simulink model "UPSControl"  (R2025b)
settings: Solver=VariableStepAuto  StartTime=0.0  StopTime=10  FixedStep=Ts  RelTol=1e-3
PostLoadFcn:
  | DataCenterParam;
values from neighbouring files (symbols this model uses):
  generator = struct    [GeneratorParam.m]
  lineInductance = 1e-6    (= 1e-06)    [DataCenterParam.m]    (also in GridParam.m)
  lineResistance = 1e-3    (= 0.001)    [DataCenterParam.m]    (also in GridParam.m)
  loadPower = 5e6    (= 5000000)    [DataCenterParam.m]    (also in LVRT.m; RedundancyAnalysis.m = 10000000)
  machine = struct    [GeneratorParam.m]
  powerTau = 0.005    [DataCenterParam.m]
  Ts = 5e-5    (= 5e-05)    [DataCenterParam.m]    (also in GeneratorParam.m)
  utilizationFactor = 0.45    [DataCenterParam.m]    (also in RedundancyAnalysis.m)
undefined symbols (not defined in the file or in its folder): breaker, ctLimitDelayTime, DiscIntNeverNeededParam, ee_sli_rtmsupport, gcbh, grid, rack, ups
libraries: nesl_utility x96, fl_lib x96, eeGeneralControl x84, ee_lib x80, simulink x68, eeTransforms x30, nesl_utility_internal x16, eeSinusoidalMeasurementV2 x13, slpidlib x12, simulink_extras x12, datacenter_lib x5, batteryecm_lib x4
(part 13 of 13)

== stateflow chart UPSControl/Server Load/UPS Units/Three UPS Parallel/UPS3/DC-Link/BESS/DC-DC Converter Controller/Mode Control/BMS ==
  state Discharge
    entry :
    mode = 4;
    if VPCC <= 0.1
    droopMode = 0;
    else
    droopMode = 1;
    end
    during:
    if VPCC <= 0.1
    droopMode = 0;
    else
    droopMode = 1;
    end
    vOut = Vdc/VdcRated;
    iRef = 0;
    flagCVChrg =  breakerStatus <=0 && VBatt >= VMaxBatt && abs(iBatt) < iBattTh && VPCC >= 0.8;
    flagCCChrg = breakerStatus <=0 && VBatt <= VMaxBatt && abs(iBatt) < iBattTh && VPCC >= 0.8;
  state Stand_by
    entry :
    mode = initialMode;
  state Float_Charging
    entry :
    mode = 3;
    during:
    vOut = VMaxBatt/VBattNom;
    iRef = 0;
    flagFloatDchrg = iPFC <= iThreshold || Vdc <= VMaxDC...
    || VPCC <= vThreshold;
  state Constant_Voltage_Charging
    entry :
    mode = 2;
    during:
    vOut = 1;
    iRef = 0;
    flagCVDchrg = (iPFC <= iThreshold || Vdc <= VMaxDC) || VPCC <= vThreshold
  state Constant_Current_Charging
    entry :
    mode = 1;
    during:
    vOut = 1;
    iRef = iCharg;
    flagCCDchrg = (iPFC <= iThreshold || Vdc <= VMaxDC) || VPCC <= vThreshold;
  (default) -> Stand_by
  Stand_by -> (junction 521) : [after(1,sec)]
  Float_Charging -> (junction 571) : [duration(flagFloatDchrg, sec) > 0.01]
  (junction 521) -> Discharge [order 1] : [mode == 4]
  (junction 521) -> Float_Charging [order 2] : [SOC >= 0.98]
  (junction 571) -> (junction 573)
  (junction 521) -> (junction 522) [order 3]
  (junction 577) -> Discharge
  (junction 575) -> (junction 577)
  (junction 566) -> Discharge
  Discharge -> (junction 524) [order 2]
  Discharge -> (junction 523) [order 1]
  (junction 580) -> Discharge
  Constant_Voltage_Charging -> Float_Charging [order 1] : [SOC >= 0.98]
  Constant_Voltage_Charging -> (junction 546) [order 2] : [duration(flagCVDchrg, sec) > 0.01]
  (junction 546) -> (junction 548)
  (junction 522) -> Constant_Voltage_Charging [order 1] : [SOC <= 0.98 && VBatt >=VMaxBatt]
  (junction 525) -> Constant_Voltage_Charging
  (junction 522) -> (junction 531) [order 2]
  (junction 527) -> (junction 525) : [duration(flagCVChrg >0 ,sec)>0.01]
  Constant_Current_Charging -> Constant_Voltage_Charging [order 1] : [VBatt >= VMaxBatt]
  (junction 531) -> Constant_Current_Charging : [SOC <=0.98 && VBatt <= VMaxBatt]
  Constant_Current_Charging -> (junction 580) [order 2] : [duration(flagCCDchrg,sec)>0.5]
  (junction 523) -> Constant_Current_Charging : [duration(flagCCChrg ,sec) > 0.5]
  (junction 524) -> (junction 527)
  (junction 548) -> (junction 566)
  (junction 573) -> (junction 575)
  data: iPFC input double; iThreshold parameter double; Vdc input double; VMaxBatt parameter double; VMaxDC parameter double; mode output double; VBatt input double =400; SOC input double; initialMode parameter; breakerStatus input; VBattNom parameter; vThreshold parameter; VPCC input; iCharg input; iRef output; vOut output; VdcRated parameter; flagCVChrg local boolean =0; flagCCDchrg local boolean =0; flagCVDchrg local boolean =0; flagFloatDchrg local boolean =0; flagCCChrg local boolean =0; iBatt input; iBattTh parameter; droopMode output

== stateflow chart UPSControl/Server Load/UPS Units/Single UPS/UPS/DC-Link/BESS/DC-DC Converter Controller/Mode Control/BMS ==
  state Discharge
    entry :
    mode = 4;
    if VPCC <= 0.1
    droopMode = 0;
    else
    droopMode = 1;
    end
    during:
    if VPCC <= 0.1
    droopMode = 0;
    else
    droopMode = 1;
    end
    vOut = Vdc/VdcRated;
    iRef = 0;
    flagCVChrg =  breakerStatus <=0 && VBatt >= VMaxBatt && abs(iBatt) < iBattTh && VPCC >= 0.8;
    flagCCChrg = breakerStatus <=0 && VBatt <= VMaxBatt && abs(iBatt) < iBattTh && VPCC >= 0.8;
  state Stand_by
    entry :
    mode = initialMode;
  state Float_Charging
    entry :
    mode = 3;
    during:
    vOut = VMaxBatt/VBattNom;
    iRef = 0;
    flagFloatDchrg = iPFC <= iThreshold || Vdc <= VMaxDC...
    || VPCC <= vThreshold;
  state Constant_Voltage_Charging
    entry :
    mode = 2;
    during:
    vOut = 1;
    iRef = 0;
    flagCVDchrg = (iPFC <= iThreshold || Vdc <= VMaxDC) || VPCC <= vThreshold
  state Constant_Current_Charging
    entry :
    mode = 1;
    during:
    vOut = 1;
    iRef = iCharg;
    flagCCDchrg = (iPFC <= iThreshold || Vdc <= VMaxDC) || VPCC <= vThreshold;
  (default) -> Stand_by
  Stand_by -> (junction 521) : [after(1,sec)]
  Float_Charging -> (junction 571) : [duration(flagFloatDchrg, sec) > 0.01]
  (junction 521) -> Discharge [order 1] : [mode == 4]
  (junction 521) -> Float_Charging [order 2] : [SOC >= 0.98]
  (junction 571) -> (junction 573)
  (junction 521) -> (junction 522) [order 3]
  (junction 577) -> Discharge
  (junction 575) -> (junction 577)
  (junction 566) -> Discharge
  Discharge -> (junction 524) [order 2]
  Discharge -> (junction 523) [order 1]
  (junction 580) -> Discharge
  Constant_Voltage_Charging -> Float_Charging [order 1] : [SOC >= 0.98]
  Constant_Voltage_Charging -> (junction 546) [order 2] : [duration(flagCVDchrg, sec) > 0.01]
  (junction 546) -> (junction 548)
  (junction 522) -> Constant_Voltage_Charging [order 1] : [SOC <= 0.98 && VBatt >=VMaxBatt]
  (junction 525) -> Constant_Voltage_Charging
  (junction 522) -> (junction 531) [order 2]
  (junction 527) -> (junction 525) : [duration(flagCVChrg >0 ,sec)>0.01]
  Constant_Current_Charging -> Constant_Voltage_Charging [order 1] : [VBatt >= VMaxBatt]
  (junction 531) -> Constant_Current_Charging : [SOC <=0.98 && VBatt <= VMaxBatt]
  Constant_Current_Charging -> (junction 580) [order 2] : [duration(flagCCDchrg,sec)>0.5]
  (junction 523) -> Constant_Current_Charging : [duration(flagCCChrg ,sec) > 0.5]
  (junction 524) -> (junction 527)
  (junction 548) -> (junction 566)
  (junction 573) -> (junction 575)
  data: iPFC input double; iThreshold parameter double; Vdc input double; VMaxBatt parameter double; VMaxDC parameter double; mode output double; VBatt input double =400; SOC input double; initialMode parameter; breakerStatus input; VBattNom parameter; vThreshold parameter; VPCC input; iCharg input; iRef output; vOut output; VdcRated parameter; flagCVChrg local boolean =0; flagCCDchrg local boolean =0; flagCVDchrg local boolean =0; flagFloatDchrg local boolean =0; flagCCChrg local boolean =0; iBatt input; iBattTh parameter; droopMode output
